simulink model "filter"  (R2021a)
settings: Solver=VariableStepAuto  StartTime=0.0  StopTime=10  RelTol=1e-3
undefined symbols (not defined in the file): Alpha, W1, W2
libraries: simulink x1
settings Model: Creator=Beshary  LastModifiedBy=Beshary

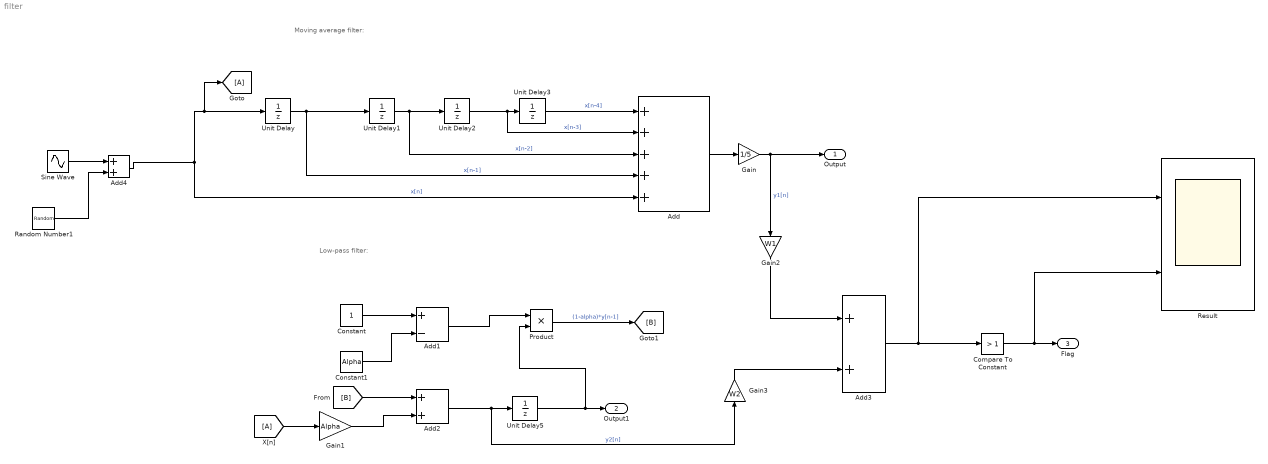
== system filter ==
  note: Low-pass filter:
  note: Moving average filter:
  Add : Sum  Inputs=+++++
  Add1 : Sum  Inputs=+-
  Add2 : Sum
  Add3 : Sum
  Add4 : Sum
  Compare To Constant : simulink/Logic and Bit Operations/Compare To Constant  relop=>  const=1  OutDataTypeStr=boolean
  Constant : Constant
  Constant1 : Constant  Value=Alpha
  Gain : Gain  Gain=1/5
  Gain1 : Gain  Gain=Alpha
  Gain2 : Gain  Gain=W1
  Gain3 : Gain  Gain=W2
  Product : Product
  Random Number1 : RandomNumber  Variance=0.01  SampleTime=0.1
  Result : Scope  NumInputPorts=2
  Sine Wave : Sin  SampleTime=0
  Unit Delay{,1..3,5} (5 alike) : UnitDelay  SampleTime=-1  HasFrameUpgradeWarning=on
  Output : Outport
  Output1 : Outport  Port=2
  Flag : Outport  Port=3
  wires:
  Unit Delay3/1 -> Add/1  "x[n-4]"
  Unit Delay2/1 -> Add/2, Unit Delay3/1  "x[n-3]"
  Unit Delay1/1 -> Add/3, Unit Delay2/1  "x[n-2]"
  Unit Delay/1 -> Add/4, Unit Delay1/1  "x[n-1]"
  Add4/1 -> [A], Unit Delay/1, Add/5  "x[n]"
  Add/1 -> Gain/1
  Gain/1 -> Gain2/1, Output/1  "y1[n]"
  Constant/1 -> Add1/1
  Constant1/1 -> Add1/2
  [A] -> Gain1/1
  Gain1/1 -> Add2/2
  Add2/1 -> Gain3/1, Unit Delay5/1  "y2[n]"
  Unit Delay5/1 -> Product/2, Output1/1
  Add1/1 -> Product/1
  Product/1 -> [B]  "(1-alpha)*y[n-1]"
  [B] -> Add2/1
  Gain2/1 -> Add3/1
  Gain3/1 -> Add3/2
  Add3/1 -> Result/1, Compare To Constant/1
  Compare To Constant/1 -> Result/2, Flag/1
  Sine Wave/1 -> Add4/1
  Random Number1/1 -> Add4/2
